simulink model "FinalModel"  (R2023b)
settings: Solver=FixedStepAuto  StartTime=0.0  StopTime=inf  RelTol=1e-3
libraries: vexarmcortexlib x28, simulink_extras x4, vexcommonlib x2
(part 2 of 2)

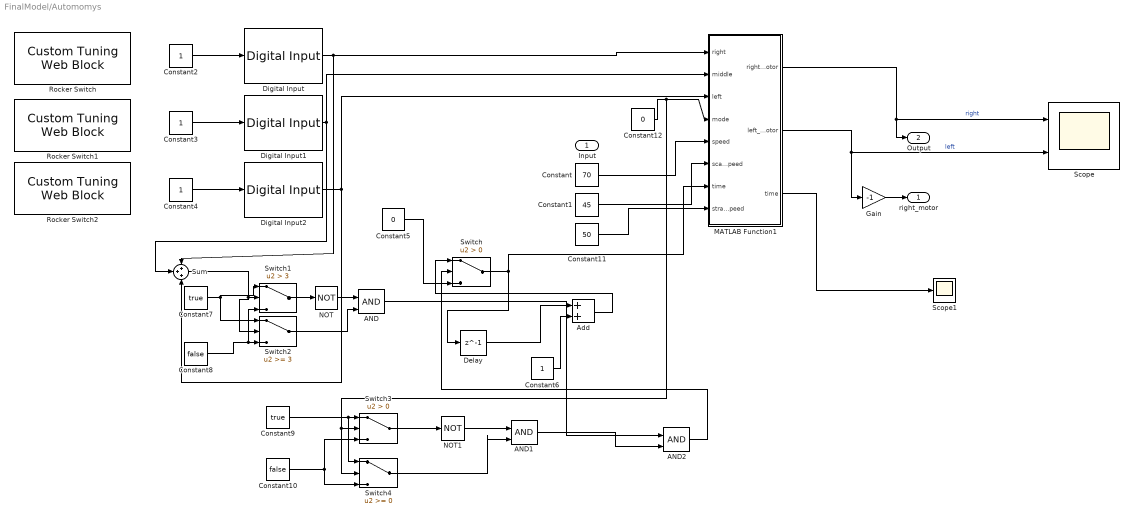
== system FinalModel/Automomys ==
  Input : Inport
  AND : Logic  IconShape=distinctive  AllPortsSameDT=off  OutDataTypeStr=boolean
  AND1 : Logic  IconShape=distinctive  AllPortsSameDT=off  OutDataTypeStr=boolean
  AND2 : Logic  IconShape=distinctive  AllPortsSameDT=off  OutDataTypeStr=boolean
  Add : Sum
  Constant : Constant  Value=70
  Constant1 : Constant  Value=45
  Constant10 : Constant  Value=false
  Constant11 : Constant  Value=50
  Constant12 : Constant  Value=0
  Constant{2..4,6} (4 alike) : Constant
  Constant5 : Constant  Value=0
  Constant7 : Constant  Value=true
  Constant8 : Constant  Value=false
  Constant9 : Constant  Value=true
  Delay : Delay  DelayLength=1
  Digital Input : vexarmcortexlib/Sensors/Digital Input  inChan=1  SimulationIn=on  SampleTime=0.2
  Digital Input1 : vexarmcortexlib/Sensors/Digital Input  inChan=2  SimulationIn=on  SampleTime=0.2
  Digital Input2 : vexarmcortexlib/Sensors/Digital Input  inChan=3  SimulationIn=on  SampleTime=0.2
  Gain : Gain  Gain=-1
  MATLAB Function1 : MATLAB Function  TreatAsAtomicUnit=on
  NOT : Logic  Operator=NOT  IconShape=distinctive  AllPortsSameDT=off  OutDataTypeStr=boolean
  NOT1 : Logic  Operator=NOT  IconShape=distinctive  AllPortsSameDT=off  OutDataTypeStr=boolean
  Rocker Switch : CustomTuningWebBlock  LabelPosition=Hide  ShowInitialText=on  Configuration="{\"components\":[{\"name\":\"CustomSwitchStateComponent\",\"settings\":{\"position\":[0,0,1,1],\"states\":[{\"HitRegion\":{\"position\":[0,0,0.5,1]},\"Image\":{\"position\":[0.13,0,1,0.75],\"size\":[1,0.75],\"src\":\"data:image\\/svg+xml;base64,PHN2ZyB4bWxucz0iaHR0cDovL3d3dy53My5vcmcvMjAwMC9zdmciIHhtbG5zOnhsaW5rPSJodHRwOi8vd3d3LnczLm9yZy8xOTk5L3hsaW5rIiB2aWV3Qm94PSIwIDAgNzUgMjQuOCI+PGRlZnM+PHN0eWxlPi5jbHMtMXtmaWxsOnVybCgjcmFkaWFsLWdyYWRpZW50KTt9LmNscy0ye2ZpbGw6dXJsKCNyYWRpYWwtZ3JhZGllbnQtMik7fS5jbHMtM3tzdHJva2U6I2IyMDAwMDtzdHJva2Utd2lkdGg6MC4yNXB4O2ZpbGw6dXJsKCNsaW5lYXItZ3JhZGllbnQpO30uY2xzLTR7ZmlsbDp1cmwoI2xpbmVhci1ncmFkaWVudC0yKTt9LmNs ...(+3576 chars)\",\"srcOrientation\":\"Right\"},\"Label\":{\"color\":[0.5019607843137255,0.5019607843137255,0.5019607843137255],\"icon\":{\"size\":[0,0],\"src\":[],\"srcOrientation\":\"Right\"},\"iconPlacement\":\"left\",\"opacity\":1,\"position\":[0.5,0.08],\"show\":true,\"text\":{\"content\":\"Off\",\"font\":\"Helvetica\",\"fontSize\":7.625366}},\"Value\":0},{\"HitRegion\":{\"position\":[0,0.5,0.5,1]},\"Image\":{\"position\":[0.13,0,1,0.75],\"size\":[1,0.75],\"src\":\"data:image\\/svg+xml;base64,PHN2ZyB4bWxucz0iaHR0cDovL3d3dy53My5vcmcvMjAwMC9zdmciIHhtbG5zOnhsaW5rPSJodHRwOi8vd3d3LnczLm9yZy8xOTk5L3hsaW5rIiB2aWV3Qm94PSIwIDAgNzUgMjQuOCI+PGRlZnM+PHN0eWxlPi5jbHMtMXtmaWxsOnVybCgjcmFkaWFsLWdyYWRpZW50KTt9LmNscy0ye2ZpbGw6dXJsKCNyYWRpYWwtZ3JhZGllbnQtMik7fS5jbHMtM3tzdHJva2U6I2IyMDAwMDtzdHJva2Utd2lkdGg6MC4yNXB4O2ZpbGw6dXJsKCNsaW5lYXItZ3JhZGllbnQpO30uY2xzLTR7ZmlsbDp1cmwoI2xpbmVhci1ncmFkaWVudC0yKTt9LmNs ...(+3520 chars)\",\"srcOrientation\":\"Right\"},\"Label\":{\"color\":[0.5019607843137255,0.5019607843137255,0.5019607843137255],\"icon\":{\"size\":[0,0],\"src\":[],\"srcOrientation\":\"Right\"},\"iconPlacement\":\"left\",\"opacity\":1,\"position\":[0.5,0.92],\"show\":true,\"text\":{\"content\":\"On\",\"font\":\"Helvetica\",\"fontSize\":7.625366}},\"Value\":1}]}},{\"name\":\"BackgroundImageComponent\",\"settings\":{\"image\":{\"size\":[155,70],\"src\":\"default\",\"srcOrientation\":\"Right\"},\"position\":[0,0,1,1],\"scaleMode\":\"0\"}},{\"name\":\"ForegroundImageComponent\",\"settings\":{\"image\":{\"size\":[0,0],\"src\":\"default\",\"srcOrientation\":[]},\"isForeground\":1,\"position\":[0,0,1,1],\"scaleMode\":\"0\"}}],\"settings\":{\"BindingType\":\"param\",\"backgroundColor\":[0,0,255,\"1\"],\"backgroundOffset\":0.14,\"fixedAspectRatio\":\"on\",\"foregroundColor\":[234,234,234],\"showBackgroundColor\":false,\"variant\":\"rocker\",\"version\":\"R2023a\"},\"type\":\"Switch\"}"
  Rocker Switch1 : CustomTuningWebBlock  LabelPosition=Hide  ShowInitialText=on  Configuration="{\"components\":[{\"name\":\"CustomSwitchStateComponent\",\"settings\":{\"position\":[0,0,1,1],\"states\":[{\"HitRegion\":{\"position\":[0,0,0.5,1]},\"Image\":{\"position\":[0.13,0,1,0.75],\"size\":[1,0.75],\"src\":\"data:image\\/svg+xml;base64,PHN2ZyB4bWxucz0iaHR0cDovL3d3dy53My5vcmcvMjAwMC9zdmciIHhtbG5zOnhsaW5rPSJodHRwOi8vd3d3LnczLm9yZy8xOTk5L3hsaW5rIiB2aWV3Qm94PSIwIDAgNzUgMjQuOCI+PGRlZnM+PHN0eWxlPi5jbHMtMXtmaWxsOnVybCgjcmFkaWFsLWdyYWRpZW50KTt9LmNscy0ye2ZpbGw6dXJsKCNyYWRpYWwtZ3JhZGllbnQtMik7fS5jbHMtM3tzdHJva2U6I2IyMDAwMDtzdHJva2Utd2lkdGg6MC4yNXB4O2ZpbGw6dXJsKCNsaW5lYXItZ3JhZGllbnQpO30uY2xzLTR7ZmlsbDp1cmwoI2xpbmVhci1ncmFkaWVudC0yKTt9LmNs ...(+3576 chars)\",\"srcOrientation\":\"Right\"},\"Label\":{\"color\":[0.5019607843137255,0.5019607843137255,0.5019607843137255],\"icon\":{\"size\":[0,0],\"src\":[],\"srcOrientation\":\"Right\"},\"iconPlacement\":\"left\",\"opacity\":1,\"position\":[0.5,0.08],\"show\":true,\"text\":{\"content\":\"Off\",\"font\":\"Helvetica\",\"fontSize\":7.625366}},\"Value\":0},{\"HitRegion\":{\"position\":[0,0.5,0.5,1]},\"Image\":{\"position\":[0.13,0,1,0.75],\"size\":[1,0.75],\"src\":\"data:image\\/svg+xml;base64,PHN2ZyB4bWxucz0iaHR0cDovL3d3dy53My5vcmcvMjAwMC9zdmciIHhtbG5zOnhsaW5rPSJodHRwOi8vd3d3LnczLm9yZy8xOTk5L3hsaW5rIiB2aWV3Qm94PSIwIDAgNzUgMjQuOCI+PGRlZnM+PHN0eWxlPi5jbHMtMXtmaWxsOnVybCgjcmFkaWFsLWdyYWRpZW50KTt9LmNscy0ye2ZpbGw6dXJsKCNyYWRpYWwtZ3JhZGllbnQtMik7fS5jbHMtM3tzdHJva2U6I2IyMDAwMDtzdHJva2Utd2lkdGg6MC4yNXB4O2ZpbGw6dXJsKCNsaW5lYXItZ3JhZGllbnQpO30uY2xzLTR7ZmlsbDp1cmwoI2xpbmVhci1ncmFkaWVudC0yKTt9LmNs ...(+3520 chars)\",\"srcOrientation\":\"Right\"},\"Label\":{\"color\":[0.5019607843137255,0.5019607843137255,0.5019607843137255],\"icon\":{\"size\":[0,0],\"src\":[],\"srcOrientation\":\"Right\"},\"iconPlacement\":\"left\",\"opacity\":1,\"position\":[0.5,0.92],\"show\":true,\"text\":{\"content\":\"On\",\"font\":\"Helvetica\",\"fontSize\":7.625366}},\"Value\":1}]}},{\"name\":\"BackgroundImageComponent\",\"settings\":{\"image\":{\"size\":[155,70],\"src\":\"default\",\"srcOrientation\":\"Right\"},\"position\":[0,0,1,1],\"scaleMode\":\"0\"}},{\"name\":\"ForegroundImageComponent\",\"settings\":{\"image\":{\"size\":[0,0],\"src\":\"default\",\"srcOrientation\":[]},\"isForeground\":1,\"position\":[0,0,1,1],\"scaleMode\":\"0\"}}],\"settings\":{\"BindingType\":\"param\",\"backgroundColor\":[0,0,255,\"1\"],\"backgroundOffset\":0.14,\"fixedAspectRatio\":\"on\",\"foregroundColor\":[234,234,234],\"showBackgroundColor\":false,\"variant\":\"rocker\",\"version\":\"R2023a\"},\"type\":\"Switch\"}"
  Rocker Switch2 : CustomTuningWebBlock  LabelPosition=Hide  ShowInitialText=on  Configuration="{\"components\":[{\"name\":\"CustomSwitchStateComponent\",\"settings\":{\"position\":[0,0,1,1],\"states\":[{\"HitRegion\":{\"position\":[0,0,0.5,1]},\"Image\":{\"position\":[0.13,0,1,0.75],\"size\":[1,0.75],\"src\":\"data:image\\/svg+xml;base64,PHN2ZyB4bWxucz0iaHR0cDovL3d3dy53My5vcmcvMjAwMC9zdmciIHhtbG5zOnhsaW5rPSJodHRwOi8vd3d3LnczLm9yZy8xOTk5L3hsaW5rIiB2aWV3Qm94PSIwIDAgNzUgMjQuOCI+PGRlZnM+PHN0eWxlPi5jbHMtMXtmaWxsOnVybCgjcmFkaWFsLWdyYWRpZW50KTt9LmNscy0ye2ZpbGw6dXJsKCNyYWRpYWwtZ3JhZGllbnQtMik7fS5jbHMtM3tzdHJva2U6I2IyMDAwMDtzdHJva2Utd2lkdGg6MC4yNXB4O2ZpbGw6dXJsKCNsaW5lYXItZ3JhZGllbnQpO30uY2xzLTR7ZmlsbDp1cmwoI2xpbmVhci1ncmFkaWVudC0yKTt9LmNs ...(+3576 chars)\",\"srcOrientation\":\"Right\"},\"Label\":{\"color\":[0.5019607843137255,0.5019607843137255,0.5019607843137255],\"icon\":{\"size\":[0,0],\"src\":[],\"srcOrientation\":\"Right\"},\"iconPlacement\":\"left\",\"opacity\":1,\"position\":[0.5,0.08],\"show\":true,\"text\":{\"content\":\"Off\",\"font\":\"Helvetica\",\"fontSize\":7.625366}},\"Value\":0},{\"HitRegion\":{\"position\":[0,0.5,0.5,1]},\"Image\":{\"position\":[0.13,0,1,0.75],\"size\":[1,0.75],\"src\":\"data:image\\/svg+xml;base64,PHN2ZyB4bWxucz0iaHR0cDovL3d3dy53My5vcmcvMjAwMC9zdmciIHhtbG5zOnhsaW5rPSJodHRwOi8vd3d3LnczLm9yZy8xOTk5L3hsaW5rIiB2aWV3Qm94PSIwIDAgNzUgMjQuOCI+PGRlZnM+PHN0eWxlPi5jbHMtMXtmaWxsOnVybCgjcmFkaWFsLWdyYWRpZW50KTt9LmNscy0ye2ZpbGw6dXJsKCNyYWRpYWwtZ3JhZGllbnQtMik7fS5jbHMtM3tzdHJva2U6I2IyMDAwMDtzdHJva2Utd2lkdGg6MC4yNXB4O2ZpbGw6dXJsKCNsaW5lYXItZ3JhZGllbnQpO30uY2xzLTR7ZmlsbDp1cmwoI2xpbmVhci1ncmFkaWVudC0yKTt9LmNs ...(+3520 chars)\",\"srcOrientation\":\"Right\"},\"Label\":{\"color\":[0.5019607843137255,0.5019607843137255,0.5019607843137255],\"icon\":{\"size\":[0,0],\"src\":[],\"srcOrientation\":\"Right\"},\"iconPlacement\":\"left\",\"opacity\":1,\"position\":[0.5,0.92],\"show\":true,\"text\":{\"content\":\"On\",\"font\":\"Helvetica\",\"fontSize\":7.625366}},\"Value\":1}]}},{\"name\":\"BackgroundImageComponent\",\"settings\":{\"image\":{\"size\":[155,70],\"src\":\"default\",\"srcOrientation\":\"Right\"},\"position\":[0,0,1,1],\"scaleMode\":\"0\"}},{\"name\":\"ForegroundImageComponent\",\"settings\":{\"image\":{\"size\":[0,0],\"src\":\"default\",\"srcOrientation\":[]},\"isForeground\":1,\"position\":[0,0,1,1],\"scaleMode\":\"0\"}}],\"settings\":{\"BindingType\":\"param\",\"backgroundColor\":[0,0,255,\"1\"],\"backgroundOffset\":0.14,\"fixedAspectRatio\":\"on\",\"foregroundColor\":[234,234,234],\"showBackgroundColor\":false,\"variant\":\"rocker\",\"version\":\"R2023a\"},\"type\":\"Switch\"}"
  Scope : Scope  NumInputPorts=2
  Scope1 : Scope
  Sum : Sum  Inputs=+++
  Switch : Switch  Criteria=u2 > Threshold  SaturateOnIntegerOverflow=off  InputSameDT=off
  Switch1 : Switch  Criteria=u2 > Threshold  Threshold=3  SaturateOnIntegerOverflow=off  InputSameDT=off
  Switch2 : Switch  Threshold=3  SaturateOnIntegerOverflow=off  InputSameDT=off
  Switch3 : Switch  Criteria=u2 > Threshold  SaturateOnIntegerOverflow=off  InputSameDT=off
  Switch4 : Switch  SaturateOnIntegerOverflow=off  InputSameDT=off
  right_motor : Outport
  Output : Outport  Port=2
  wires:
  MATLAB Function1/2(left_motor) -> Gain/1, Scope/2  "left"
  MATLAB Function1/1(right_motor) -> Output/1, Scope/1  "right"
  Digital Input2/1 -> Sum/3, MATLAB Function1/3(left)
  Digital Input1/1 -> Sum/2, MATLAB Function1/2(middle)
  Digital Input/1 -> Sum/1, MATLAB Function1/1(right)
  Constant12/1 -> Switch4/2, Switch3/2, MATLAB Function1/4(mode)
  Constant/1 -> MATLAB Function1/5(speed)
  Constant1/1 -> MATLAB Function1/6(scanspeed)
  Constant2/1 -> Digital Input/1
  Constant3/1 -> Digital Input1/1
  Constant4/1 -> Digital Input2/1
  Switch/1 -> MATLAB Function1/7("time "), Delay/1
  Delay/1 -> Add/1
  Constant6/1 -> Add/2
  Sum/1 -> Switch2/2, Switch1/2
  Switch1/1 -> NOT/1
  NOT/1 -> AND/1
  Switch2/1 -> AND/2
  Constant8/1 -> Switch1/3, Switch2/3
  Constant7/1 -> Switch2/1, Switch1/1
  Add/1 -> Switch/1
  Constant5/1 -> Switch/3
  Gain/1 -> right_motor/1
  Constant10/1 -> Switch3/3, Switch4/3
  Constant9/1 -> Switch4/1, Switch3/1
  Switch3/1 -> NOT1/1
  NOT1/1 -> AND1/1
  Switch4/1 -> AND1/2
  AND2/1 -> Switch/2
  AND/1 -> AND2/1
  AND1/1 -> AND2/2
  Constant11/1 -> MATLAB Function1/8(straightspeed)
  MATLAB Function1/3(time) -> Scope1/1

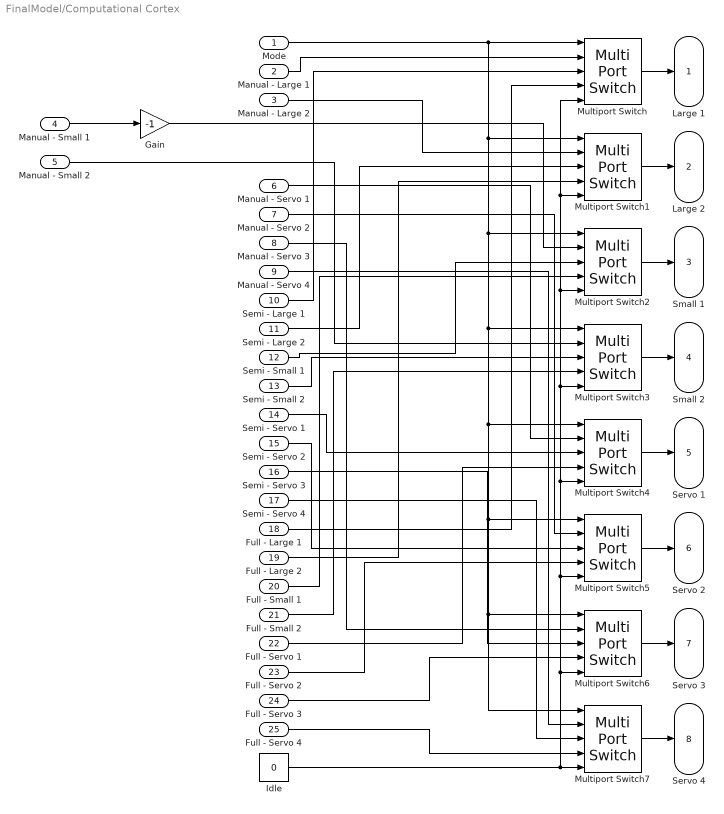
== system FinalModel/Computational Cortex ==
  Mode : Inport
  Manual - Large 1 : Inport  Port=2
  Manual - Large 2 : Inport  Port=3
  Manual - Small 1 : Inport  Port=4
  Manual - Small 2 : Inport  Port=5
  Manual - Servo 1 : Inport  Port=6
  Manual - Servo 2 : Inport  Port=7
  Manual - Servo 3 : Inport  Port=8
  Manual - Servo 4 : Inport  Port=9
  Semi - Large 1 : Inport  Port=10
  Semi - Large 2 : Inport  Port=11
  Semi - Small 1 : Inport  Port=12
  Semi - Small 2 : Inport  Port=13
  Semi - Servo 1 : Inport  Port=14
  Semi - Servo 2 : Inport  Port=15
  Semi - Servo 3 : Inport  Port=16
  Semi - Servo 4 : Inport  Port=17
  Full - Large 1 : Inport  Port=18
  Full - Large 2 : Inport  Port=19
  Full - Small 1 : Inport  Port=20
  Full - Small 2 : Inport  Port=21
  Full - Servo 1 : Inport  Port=22
  Full - Servo 2 : Inport  Port=23
  Full - Servo 3 : Inport  Port=24
  Full - Servo 4 : Inport  Port=25
  Gain : Gain  Gain=-1
  Idle : Constant  Value=0
  Multiport Switch{,1..7} (8 alike) : MultiPortSwitch  Inputs=4  SaturateOnIntegerOverflow=off  InputSameDT=off
  Large 1 : Outport
  Large 2 : Outport  Port=2
  Small 1 : Outport  Port=3
  Small 2 : Outport  Port=4
  Servo 1 : Outport  Port=5
  Servo 2 : Outport  Port=6
  Servo 3 : Outport  Port=7
  Servo 4 : Outport  Port=8
  wires:
  Multiport Switch/1 -> Large 1/1
  Multiport Switch1/1 -> Large 2/1
  Multiport Switch3/1 -> Small 2/1
  Multiport Switch2/1 -> Small 1/1
  Multiport Switch5/1 -> Servo 2/1
  Multiport Switch4/1 -> Servo 1/1
  Multiport Switch7/1 -> Servo 4/1
  Multiport Switch6/1 -> Servo 3/1
  Idle/1 -> Multiport Switch/5, Multiport Switch1/5, Multiport Switch2/5, Multiport Switch3/5, Multiport Switch4/5, Multiport Switch5/5, Multiport Switch6/5, Multiport Switch7/5
  Full - Servo 4/1 -> Multiport Switch7/4
  Full - Servo 3/1 -> Multiport Switch6/4
  Full - Servo 2/1 -> Multiport Switch5/4
  Full - Servo 1/1 -> Multiport Switch4/4
  Full - Small 2/1 -> Multiport Switch3/4
  Full - Small 1/1 -> Multiport Switch2/4
  Full - Large 2/1 -> Multiport Switch1/4
  Full - Large 1/1 -> Multiport Switch/4
  Semi - Servo 4/1 -> Multiport Switch7/3
  Semi - Servo 3/1 -> Multiport Switch6/3
  Semi - Servo 2/1 -> Multiport Switch5/3
  Semi - Servo 1/1 -> Multiport Switch4/3
  Semi - Small 2/1 -> Multiport Switch3/3
  Semi - Small 1/1 -> Multiport Switch2/3
  Semi - Large 2/1 -> Multiport Switch1/3
  Semi - Large 1/1 -> Multiport Switch/3
  Manual - Servo 4/1 -> Multiport Switch7/2
  Manual - Servo 3/1 -> Multiport Switch6/2
  Manual - Servo 2/1 -> Multiport Switch5/2
  Manual - Servo 1/1 -> Multiport Switch4/2
  Manual - Small 1/1 -> Gain/1
  Manual - Large 2/1 -> Multiport Switch1/2
  Manual - Large 1/1 -> Multiport Switch/2
  Mode/1 -> Multiport Switch3/1, Multiport Switch4/1, Multiport Switch7/1, Multiport Switch6/1, Multiport Switch5/1, Multiport Switch2/1, Multiport Switch1/1, Multiport Switch/1
  Manual - Small 2/1 -> Multiport Switch3/2
  Gain/1 -> Multiport Switch2/2

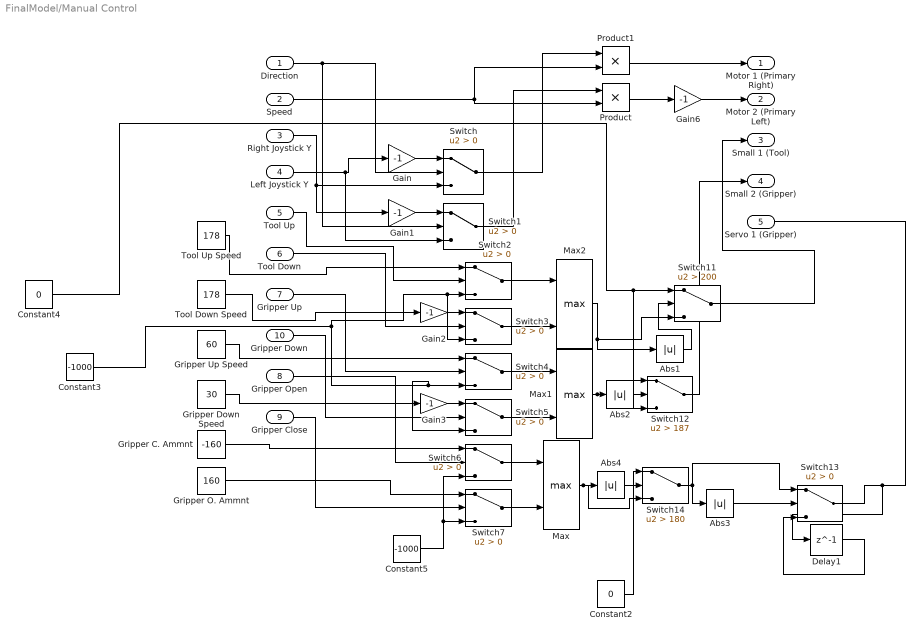
== system FinalModel/Manual Control ==
  Direction : Inport
  Speed : Inport  Port=2
  Right Joystick Y : Inport  Port=3
  Left Joystick Y : Inport  Port=4
  Tool Up : Inport  Port=5
  Tool Down : Inport  Port=6
  Gripper Up : Inport  Port=7
  Gripper Open : Inport  Port=8
  Gripper Close : Inport  Port=9
  Gripper Down : Inport  Port=10
  Abs{1..4} (4 alike) : Abs  SaturateOnIntegerOverflow=off
  Constant2 : Constant  Value=0
  Constant3 : Constant  Value=-1000
  Constant4 : Constant  Value=0
  Constant5 : Constant  Value=-1000
  Delay1 : Delay  DelayLength=1
  Gain{,1..3,6} (5 alike) : Gain  Gain=-1
  Gripper C. Ammnt : Constant  Value=-160
  Gripper Down Speed : Constant  Value=30
  Gripper O. Ammnt : Constant  Value=160
  Gripper Up Speed : Constant  Value=60
  Max : MinMax  Function=max  Inputs=2
  Max1 : MinMax  Function=max  Inputs=2
  Max2 : MinMax  Function=max  Inputs=2
  Product : Product  RndMeth=Zero
  Product1 : Product  RndMeth=Zero
  Switch{,1..7,13} (9 alike) : Switch  Criteria=u2 > Threshold  SaturateOnIntegerOverflow=off  InputSameDT=off
  Switch11 : Switch  Criteria=u2 > Threshold  Threshold=200  SaturateOnIntegerOverflow=off  InputSameDT=off
  Switch12 : Switch  Criteria=u2 > Threshold  Threshold=187  SaturateOnIntegerOverflow=off  InputSameDT=off
  Switch14 : Switch  Criteria=u2 > Threshold  Threshold=180  SaturateOnIntegerOverflow=off  InputSameDT=off
  Tool Down Speed : Constant  Value=178
  Tool Up Speed : Constant  Value=178
  Motor 1 (Primary Right) : Outport
  Motor 2 (Primary Left) : Outport  Port=2
  Small 1 (Tool) : Outport  Port=3
  Small 2 (Gripper) : Outport  Port=4
  Servo 1 (Gripper) : Outport  Port=5
  wires:
  Gripper Close/1 -> Switch7/2
  Gripper Down Speed/1 -> Gain3/1
  Constant4/1 -> Switch12/1, Switch11/1
  Direction/1 -> Switch1/2, Switch/2
  Tool Down/1 -> Switch3/2
  Delay1/1 -> Switch13/3
  Gripper C. Ammnt/1 -> Switch6/1
  Max1/1 -> Switch12/3, Abs2/1
  Abs1/1 -> Switch11/2
  Tool Down Speed/1 -> Gain2/1
  Tool Up/1 -> Switch2/2
  Abs2/1 -> Switch12/2
  Max2/1 -> Abs1/1, Switch11/3
  Gain3/1 -> Switch5/1
  Constant3/1 -> Switch3/3, Switch2/3, Switch5/3, Switch4/3
  Switch6/1 -> Max/1
  Constant2/1 -> Switch14/1
  Switch13/1 -> Delay1/1, Servo 1 (Gripper)/1
  Gain2/1 -> Switch3/1
  Left Joystick Y/1 -> Switch1/3, Gain/1
  Switch/1 -> Product1/1
  Gripper Down/1 -> Switch5/2
  Gripper Open/1 -> Switch6/2
  Tool Up Speed/1 -> Switch2/1
  Gripper Up/1 -> Switch4/2
  Switch12/1 -> Small 2 (Gripper)/1
  Switch7/1 -> Max/2
  Speed/1 -> Product/2, Product1/2
  Switch4/1 -> Max1/1
  Switch2/1 -> Max2/1
  Gripper O. Ammnt/1 -> Switch7/1
  Gripper Up Speed/1 -> Switch4/1
  Switch5/1 -> Max1/2
  Gain1/1 -> Switch1/1
  Switch3/1 -> Max2/2
  Right Joystick Y/1 -> Switch/3, Gain1/1
  Switch1/1 -> Product/1
  Gain/1 -> Switch/1
  Abs3/1 -> Switch13/2
  Constant5/1 -> Switch6/3, Switch7/3
  Max/1 -> Switch14/3, Abs4/1
  Abs4/1 -> Switch14/2
  Switch14/1 -> Abs3/1, Switch13/1
  Product/1 -> Gain6/1
  Gain6/1 -> Motor 2 (Primary Left)/1
  Product1/1 -> Motor 1 (Primary Right)/1
  Switch11/1 -> Small 1 (Tool)/1

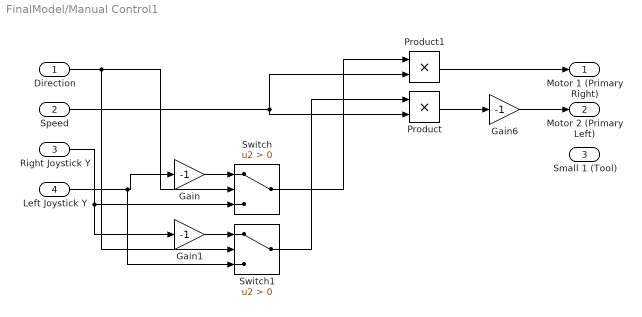
== system FinalModel/Manual Control1 ==
  Direction : Inport
  Speed : Inport  Port=2
  Right Joystick Y : Inport  Port=3
  Left Joystick Y : Inport  Port=4
  Gain : Gain  Gain=-1
  Gain1 : Gain  Gain=-1
  Gain6 : Gain  Gain=-1
  Product : Product  RndMeth=Zero
  Product1 : Product  RndMeth=Zero
  Switch : Switch  Criteria=u2 > Threshold  SaturateOnIntegerOverflow=off  InputSameDT=off
  Switch1 : Switch  Criteria=u2 > Threshold  SaturateOnIntegerOverflow=off  InputSameDT=off
  Motor 1 (Primary Right) : Outport
  Motor 2 (Primary Left) : Outport  Port=2
  Small 1 (Tool) : Outport  Port=3
  wires:
  Direction/1 -> Switch1/2, Switch/2
  Left Joystick Y/1 -> Switch1/3, Gain/1
  Switch/1 -> Product1/1
  Speed/1 -> Product/2, Product1/2
  Gain1/1 -> Switch1/1
  Right Joystick Y/1 -> Switch/3, Gain1/1
  Switch1/1 -> Product/1
  Gain/1 -> Switch/1
  Product/1 -> Gain6/1
  Gain6/1 -> Motor 2 (Primary Left)/1
  Product1/1 -> Motor 1 (Primary Right)/1

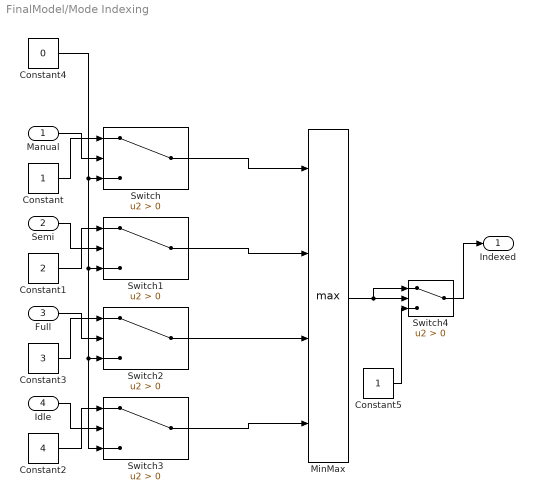
== system FinalModel/Mode Indexing ==
  Manual : Inport
  Semi : Inport  Port=2
  Full : Inport  Port=3
  Idle : Inport  Port=4
  Constant : Constant
  Constant1 : Constant  Value=2
  Constant2 : Constant  Value=4
  Constant3 : Constant  Value=3
  Constant4 : Constant  Value=0
  Constant5 : Constant
  MinMax : MinMax  Function=max  Inputs=4
  Switch{,1..4} (5 alike) : Switch  Criteria=u2 > Threshold  SaturateOnIntegerOverflow=off  InputSameDT=off
  Indexed : Outport
  wires:
  Switch/1 -> MinMax/1
  Switch1/1 -> MinMax/2
  Switch2/1 -> MinMax/3
  Switch3/1 -> MinMax/4
  Manual/1 -> Switch/2
  Constant/1 -> Switch/1
  Constant1/1 -> Switch1/1
  Semi/1 -> Switch1/2
  Full/1 -> Switch2/2
  Constant3/1 -> Switch2/1
  Constant2/1 -> Switch3/1
  Idle/1 -> Switch3/2
  Constant4/1 -> Switch3/3, Switch2/3, Switch1/3, Switch/3
  MinMax/1 -> Switch4/1, Switch4/2
  Switch4/1 -> Indexed/1
  Constant5/1 -> Switch4/3

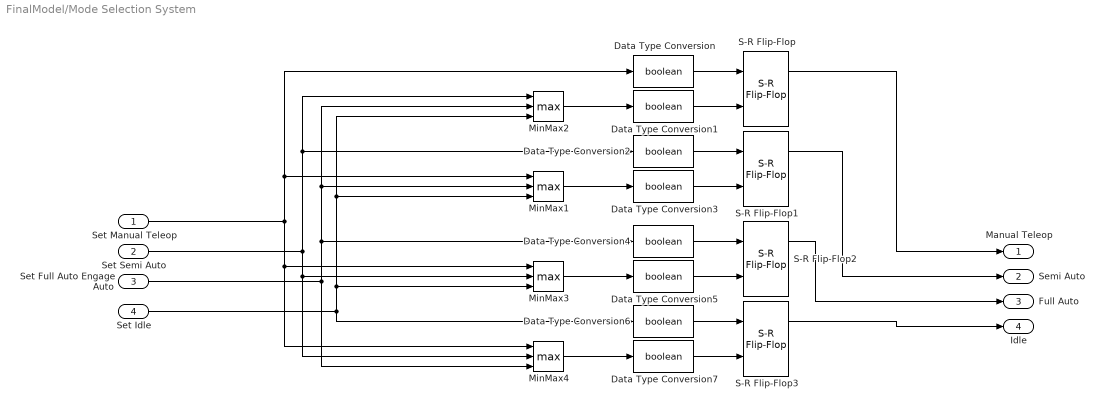
== system FinalModel/Mode Selection System ==
  Set Manual Teleop : Inport
  Set Semi Auto : Inport  Port=2
  Set Full Auto Engage Auto : Inport  Port=3
  Set Idle : Inport  Port=4
  Data Type Conversion{,1..7} (8 alike) : DataTypeConversion  OutDataTypeStr=boolean  ConvertRealWorld=Stored Integer (SI)  SaturateOnIntegerOverflow=off  RndMeth=Floor
  MinMax{1..4} (4 alike) : MinMax  Function=max  Inputs=3
  S-R Flip-Flop{,1..3} (4 alike) : simulink_extras/Flip Flops/S-R Flip-Flop  initial_condition=0
  Manual Teleop : Outport
  Semi Auto : Outport  Port=2
  Full Auto : Outport  Port=3
  Idle : Outport  Port=4
  wires:
  Set Semi Auto/1 -> MinMax3/2, MinMax4/2, MinMax2/1, Data Type Conversion2/1
  Set Full Auto Engage Auto/1 -> MinMax4/3, MinMax1/2, MinMax2/2, Data Type Conversion4/1
  Set Idle/1 -> Data Type Conversion6/1, MinMax3/3, MinMax1/3, MinMax2/3
  S-R Flip-Flop/1 -> Manual Teleop/1
  Data Type Conversion/1 -> S-R Flip-Flop/1
  Data Type Conversion1/1 -> S-R Flip-Flop/2
  MinMax2/1 -> Data Type Conversion1/1
  Set Manual Teleop/1 -> Data Type Conversion/1, MinMax1/1, MinMax3/1, MinMax4/1
  Data Type Conversion2/1 -> S-R Flip-Flop1/1
  MinMax1/1 -> Data Type Conversion3/1
  S-R Flip-Flop1/1 -> Semi Auto/1
  Data Type Conversion3/1 -> S-R Flip-Flop1/2
  Data Type Conversion4/1 -> S-R Flip-Flop2/1
  MinMax3/1 -> Data Type Conversion5/1
  S-R Flip-Flop2/1 -> Full Auto/1
  Data Type Conversion5/1 -> S-R Flip-Flop2/2
  Data Type Conversion6/1 -> S-R Flip-Flop3/1
  MinMax4/1 -> Data Type Conversion7/1
  S-R Flip-Flop3/1 -> Idle/1
  Data Type Conversion7/1 -> S-R Flip-Flop3/2

== matlab function FinalModel/Automomys/MATLAB Function1 ==
  data: right input; right_motor output; middle input; left input; mode input; speed input; scanspeed input; left_motor output; time input; straightspeed input; time output
function [right_motor, left_motor, time]  = line_follow(right, middle, left, mode, speed, scanspeed, time, straightspeed)
right_motor = 0;
left_motor = 0;
if mode == 0
   if left == 1 && middle == 0 && right == 1
       %Straight
       right_motor = straightspeed;
       left_motor = straightspeed;
   elseif left == 1 && middle == 0 && right == 0
       %RightSlight
       right_motor = speed/2;
       left_motor = speed;
   elseif left == 1 && middle == 1 && right == 0
       %Right
       right_motor = -speed/2;
       left_motor = speed/2;
   elseif left == 0 && middle == 0 && right == 1
       %LeftSlight
       right_motor = speed;
       left_motor = speed/2;
   elseif left == 0 && middle == 1 && right == 1
       %Left
       right_motor = speed/2;
       left_motor = -speed/2;
   else     %scanning
       if time < 25 %change to time off
           %scan right
           right_motor = -scanspeed;
           left_motor = scanspeed;
       elseif time >= 25 && time < 75 %change to time off
           %scan left
           right_motor = scanspeed;
           left_motor = -scanspeed;
       elseif time >= 75 && time < 100  %change to time off
           right_motor = -scanspeed;
           left_motor = scanspeed;
       elseif time >= 100 && time < 105  %change to time off
           right_motor = 0;
           left_motor = 0;           
       else
           left_motor = -scanspeed;
           right_motor = -scanspeed;
       end
   end
end
